simulink model "solics_inverter_model"  (R2024a)
settings: Solver=VariableStepAuto  StartTime=0.0  StopTime=10.0  RelTol=1e-3
libraries: fl_lib x1, rfseriesshuntrlcs1 x1, nesl_utility x1
settings Model: Creator=dogba  LastModifiedBy=dogba

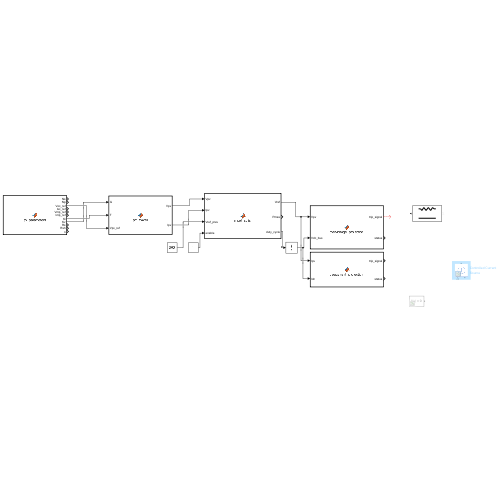
[thumbnail: Simulink's stored preview of the top-level diagram]
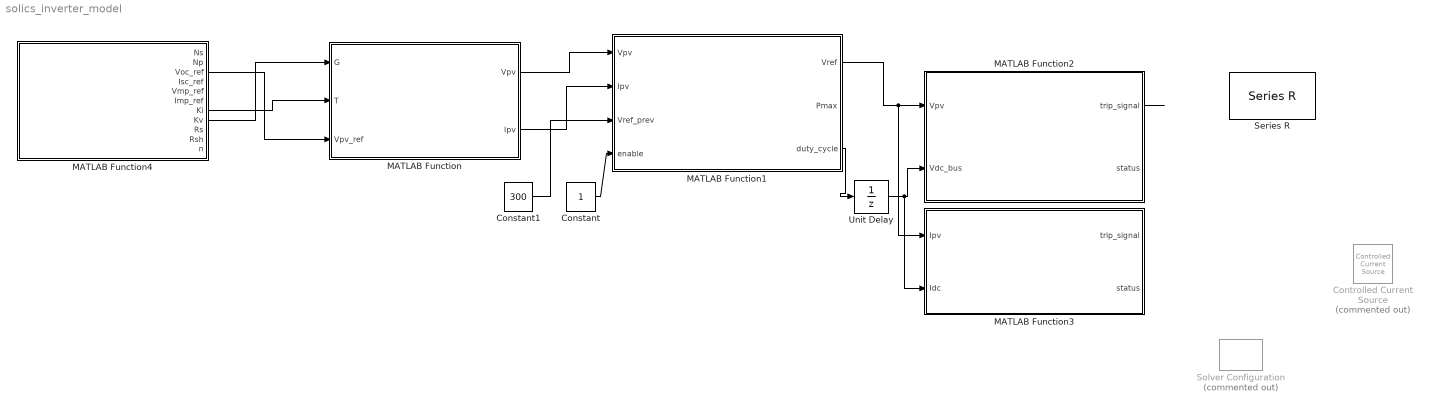
== system solics_inverter_model ==
  Constant : Constant  SampleTime=0.001
  Constant1 : Constant  Value=300  SampleTime=0.001
  Controlled Current Source : fl_lib/Electrical/Electrical Sources/Controlled Current Source  Commented=on
  MATLAB Function : MATLAB Function  TreatAsAtomicUnit=on
  MATLAB Function1 : MATLAB Function  TreatAsAtomicUnit=on
  MATLAB Function2 : MATLAB Function  TreatAsAtomicUnit=on
  MATLAB Function3 : MATLAB Function  TreatAsAtomicUnit=on
  MATLAB Function4 : MATLAB Function  TreatAsAtomicUnit=on
  Series R : rfseriesshuntrlcs1/Series R  LConnTagsString=__newl0  RConnTagsString=__newr0  R=1  L=0  C=Inf  PlotFreq=User-specified  SourceFreq=User-specified  Freq=[1:1.0e5:4e6]  AllPlotType=X-Y plane  AppliedNetworkData=S21  AppliedComplexFormat=Magnitude (decibels)  AppliedNetworkData2=""  AppliedXParameter=Freq  AppliedXFormat=Hz  YOption=Linear  XOption=Linear  PlotZ0=50  DisplayData=off  PlotFreqNoSim=User-specified  NetworkData=S21  SmithData=S11  PolarData=S11  ComplexFormat=Magnitude (decibels)  DBFormat=Magnitude (decibels)  NoneFormat=None
  Solver Configuration : nesl_utility/Solver Configuration  Commented=on  PhysicalDomain=network_engine_domain  SubClassName=solver  LeftPortType=input  RightPortType=generic  Tones=[]  Harmonics=[]  SimulateNoise=off  Profile=off  UseLocalSampling=off  EnableSwitchedLinearOptims=on  FrequencyDomain=off  UseCCode=off  RelTol=0.001  AbsTol=0.001  MinStep=1e-09  ToWorkspace=off  RevertToSquareIcSolve=off  NumHomotopyIterations=100  PhasorMode=off  PhasorModeNumHarmonics=1  ConsistencySolver=NEWTON_XTOL_AFTER_FTOL  IndexReductionMethod=DerivativeReplacement  DoDC=off  ResidualTolerance=1e-09  ConsistencyTolSource=GLOBAL  ConsistencyAbsTol=0.001  ConsistencyRelTol=0.001  ConsistencyTolFactor=0.001  UseLocalSolver=off  LocalSolverChoice=NE_BACKWARD_EULER_ADVANCER  ResolveIndetEquations=on  FunctionEvalNumThread=1  LocalSolverSampleTime=0.001  DoFixedCost=off  MaxNonlinIter=3  MaxModeIter=2  ComputeImpulses=off  ImpulseIterations=2  LinearAlgebra=auto  LinearAlgebraNumThread=0  EquationFormulation=NE_TIME_EF  DelaysMemoryBudget=1024  AutomaticFiltering=on  FilteringTimeConstant=0.001  PartitionStorageMethod=AS_NEEDED  PartitionMemoryBudget=1024  PartitionMethod=ROBUST  MultibodyUseLocalSolver=off  MultibodyLocalSolverChoice=ODE1  MultibodyLocalSolverSampleTime=0.001
  Unit Delay : UnitDelay  InitialCondition=300  SampleTime=0.001  HasFrameUpgradeWarning=on
  wires:
  MATLAB Function4/3(Voc_ref) -> MATLAB Function/3(Vpv_ref)
  MATLAB Function4/7(Ki) -> MATLAB Function/2(T)
  MATLAB Function4/8(Kv) -> MATLAB Function/1(G)
  MATLAB Function/1(Vpv) -> MATLAB Function1/1(Vpv)
  MATLAB Function/2(Ipv) -> MATLAB Function1/2(Ipv)
  Constant1/1 -> MATLAB Function1/3(Vref_prev)
  Constant/1 -> MATLAB Function1/4(enable)
  MATLAB Function1/1(Vref) -> MATLAB Function3/1(Ipv), MATLAB Function2/1(Vpv)
  MATLAB Function1/3(duty_cycle) -> Unit Delay/1
  Unit Delay/1 -> MATLAB Function3/2(Idc), MATLAB Function2/2(Vdc_bus)
  MATLAB Function2/1(trip_signal) -> ?

== matlab function solics_inverter_model/MATLAB Function1 ==
  data: Vpv input; Vref output; Ipv input; Vref_prev input; enable input; Pmax output; duty_cycle output
function [Vref, Pmax, duty_cycle] = mppt_solis(Vpv, Ipv, Vref_prev, enable)
    % Solis MPPT Algorithm (Perturb & Observe with modifications)
    persistent Ppv_prev Vpv_prev step_size direction
    
    % Initialize persistent variables
    if isempty(Ppv_prev)
        Ppv_prev = 0;
        Vpv_prev = 0;
        step_size = 0.5;  % Initial step size (V)
        direction = 1;    % Initial direction
    end
    
    % Calculate current power
    Ppv = Vpv * Ipv;
    Pmax = Ppv;
    
    % MPPT disabled condition
    if ~enable
        Vref = Vref_prev;
        duty_cycle = 0;
        return;
    end
    
    % Calculate changes
    dP = Ppv - Ppv_prev;
    dV = Vpv - Vpv_prev;
    
    % Perturb & Observe Algorithm with adaptive step size
    if abs(dP) > 0.1  % Power change threshold
        if dP > 0
            % Power increased, continue in same direction
            if dV > 0
                direction = 1;   % Increase voltage
            else
                direction = -1;  % Decrease voltage
            end
            step_size = min(step_size * 1.1, 2.0);  % Increase step size
        else
            % Power decreased, reverse direction
            direction = -direction;
            step_size = max(step_size * 0.9, 0.1);  % Decrease step size
        end
    end
    
    % Calculate new reference voltage
    Vref = Vref_prev + direction * step_size;
    
    % Voltage limits for Solis inverter
    Vref = max(min(Vref, 1000), 80);  % 80V min, 1000V max
    
    % Calculate duty cycle for boost converter
    Vdc_bus = 400;  % Target DC bus voltage
    duty_cycle = max(0, min(0.9, 1 - Vpv/Vdc_bus));
    
    % Update previous values
    Ppv_prev = Ppv;
    Vpv_prev = Vpv;
end

== matlab function solics_inverter_model/MATLAB Function ==
  data: G input; Vpv output; T input; Vpv_ref input; Ipv output
function [Vpv, Ipv] = pv_model(G, T, Vpv_ref)
    % PV Model Parameters (typical for 300W silicon module)
    Voc_ref = 37.2;      % Open circuit voltage at STC (V)
    Isc_ref = 8.95;      % Short circuit current at STC (A)
    Vmp_ref = 30.8;      % Voltage at MPP at STC (V)
    Imp_ref = 9.74;      % Current at MPP at STC (A)
    
    % Temperature coefficients
    Ki = 0.0005;         % Current temperature coefficient (A/°C)
    Kv = -0.0032;        % Voltage temperature coefficient (V/°C)
    
    % Standard Test Conditions
    G_ref = 1000;        % Reference irradiance (W/m²)
    T_ref = 25;          % Reference temperature (°C)
    
    % Calculate temperature and irradiance effects
    Isc = Isc_ref * (G/G_ref) * (1 + Ki*(T - T_ref));
    Voc = Voc_ref * (1 + Kv*(T - T_ref));
    
    % Simplified current-voltage relationship
    Rs = 0.3;            % Series resistance (Ω)
    Rsh = 1000;          % Shunt resistance (Ω)
    n = 1.3;             % Ideality factor
    
    % Constants
    q = 1.602e-19;       % Elementary charge (C)
    k = 1.381e-23;       % Boltzmann constant (J/K)
    T_K = T + 273.15;    % Temperature in Kelvin
    
    % Thermal voltage
    Vt = k * T_K / q;
    
    % Photocurrent
    Iph = Isc;
    
    % Reverse saturation current
    Io = Isc / (exp(Voc/(n*Vt)) - 1);
    
    % PV current calculation (implicit equation solved iteratively)
    Vpv = Vpv_ref;
    for i = 1:10
        Ipv = Iph - Io*(exp((Vpv + Ipv*Rs)/(n*Vt)) - 1) - (Vpv + Ipv*Rs)/Rsh;
        if abs(Ipv) < 1e-6
            break;
        end
    end
    
    % Ensure positive current
    Ipv = max(0, Ipv);
end

== matlab function solics_inverter_model/MATLAB Function2 ==
  data: Vpv input; trip_signal output; Vdc_bus input; status output
function [trip_signal, status] = overvoltage_protection(Vpv, Vdc_bus)
    % Solis inverter protection limits
    Vpv_max = 1000;      % Maximum PV voltage
    Vdc_max = 900;       % Maximum DC bus voltage
    
    if Vpv > Vpv_max || Vdc_bus > Vdc_max
        trip_signal = 1;
        status = 'OVERVOLTAGE';
    else
        trip_signal = 0;
        status = 'NORMAL';
    end
end

== matlab function solics_inverter_model/MATLAB Function3 ==
  data: Ipv input; trip_signal output; Idc input; status output
function [trip_signal, status] = overcurrent_protection(Ipv, Idc)
    % Solis inverter current limits
    Ipv_max = 32;        % Maximum PV current (A)
    Idc_max = 40;        % Maximum DC current (A)
    
    if Ipv > Ipv_max || Idc > Idc_max
        trip_signal = 1;
        status = 'OVERCURRENT';
    else
        trip_signal = 0;
        status = 'NORMAL';
    end
end

== matlab function solics_inverter_model/MATLAB Function4 ==
  data: Ns output; Np output; Voc_ref output; Isc_ref output; Vmp_ref output; Imp_ref output; Ki output; Kv output; Rs output; Rsh output; n output
function [Ns, Np, Voc_ref, Isc_ref, Vmp_ref, Imp_ref, Ki, Kv, Rs, Rsh, n] = pv_parameters()
    % Solis Compatible PV Array Configuration
    % Based on typical 300W monocrystalline silicon modules
    
    % Array Configuration
    Ns = 20;             % Number of modules in series
    Np = 2;              % Number of parallel strings
    
    % Single Module Parameters at STC (25°C, 1000W/m²)
    Voc_ref = 37.2;      % Open circuit voltage (V)
    Isc_ref = 8.95;      % Short circuit current (A)
    Vmp_ref = 30.8;      % Voltage at Maximum Power Point (V)
    Imp_ref = 9.74;      % Current at Maximum Power Point (A)
    
    % Temperature Coefficients
    Ki = 0.0005;         % Current temperature coefficient (A/°C)
    Kv = -0.0032;        % Voltage temperature coefficient (V/°C)
    
    % Circuit Parameters
    Rs = 0.3;            % Series resistance (Ω)
    Rsh = 1000;          % Shunt resistance (Ω)
    n = 1.3;             % Ideality factor
end
